simulink model "ELECTRIC_RC_AIRCRAFT_simulink"  (R2025b)
settings: Solver=FixedStepAuto  StartTime=0  StopTime=1000  FixedStep=1/30  RelTol=1e-3
values from neighbouring files (symbols this model uses):
  AoA = [-5 0 5 10 15]    [ELECTRIC_RC_AIRCRAFT.m]
  C_mq = -2*((Tail_Wing_Area/Wing_Surface_Area)*(tail_moment_arm/chord_length_tail))    (= -0.900546448087)    [ELECTRIC_RC_AIRCRAFT.m]
  C_mse = -n*(Tail_Wing_Area/Wing_Surface_Area)*(tail_moment_arm/chord_length_tail)    (= -0.351213114754)    [ELECTRIC_RC_AIRCRAFT.m]
  chord_length = 0.25    [ELECTRIC_RC_AIRCRAFT.m]
  CL = [-0.249 0.205 0.752 1.190 1.316]    [ELECTRIC_RC_AIRCRAFT.m]
  CM = [0.0550 0.0260 -0.0854 -0.1805]    [ELECTRIC_RC_AIRCRAFT.m]
  g = 9.81    [ELECTRIC_RC_AIRCRAFT.m]
  Inertia = (m/12)*(fuselage_length^2+wing_span^2)    (= 0.54883225)    [ELECTRIC_RC_AIRCRAFT.m]
  m = 1.83    [ELECTRIC_RC_AIRCRAFT.m]
  Velocity_initial = 20    [ELECTRIC_RC_AIRCRAFT.m]
  Wing_Surface_Area = 0.4575    [ELECTRIC_RC_AIRCRAFT.m]
libraries: aerolibconvert2 x4, simulink x4, slpidlib x3, aerolibfltsims x2, aerolibadyn x1, aerolibasang x1, aerolibactuator x1, aerolibbdyn x1, aerolibpropulsion2 x1
settings Model: Creator=papar  LastModifiedBy=papar

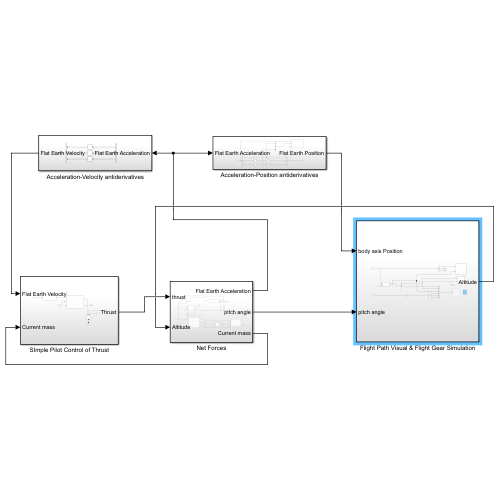
[thumbnail: Simulink's stored preview of the top-level diagram]
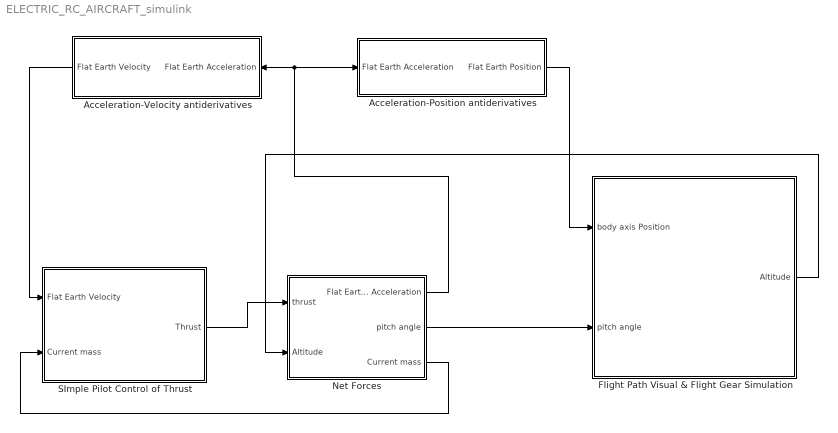
== system ELECTRIC_RC_AIRCRAFT_simulink ==
  Acceleration-Position antiderivatives : Subsystem
  Acceleration-Velocity antiderivatives : Subsystem
  Flight Path Visual & Flight Gear Simulation : Subsystem
  Net Forces : Subsystem
  SImple Pilot Control of Thrust : Subsystem
  wires:
  Acceleration-Velocity antiderivatives/1(Flat Earth Velocity) -> SImple Pilot Control of Thrust/1(Flat Earth Velocity)
  Net Forces/1(Flat Earth Acceleration) -> Acceleration-Velocity antiderivatives/1(Flat Earth Acceleration), Acceleration-Position antiderivatives/1(Flat Earth Acceleration)
  Net Forces/3(Current mass) -> SImple Pilot Control of Thrust/2(Current mass)
  SImple Pilot Control of Thrust/1(Thrust) -> Net Forces/1(thrust)
  Acceleration-Position antiderivatives/1(Flat Earth Position) -> Flight Path Visual & Flight Gear Simulation/1(body axis Position)
  Net Forces/2(pitch angle) -> Flight Path Visual & Flight Gear Simulation/2(pitch angle)
  Flight Path Visual & Flight Gear Simulation/1(Altitude) -> Net Forces/2(Altitude)

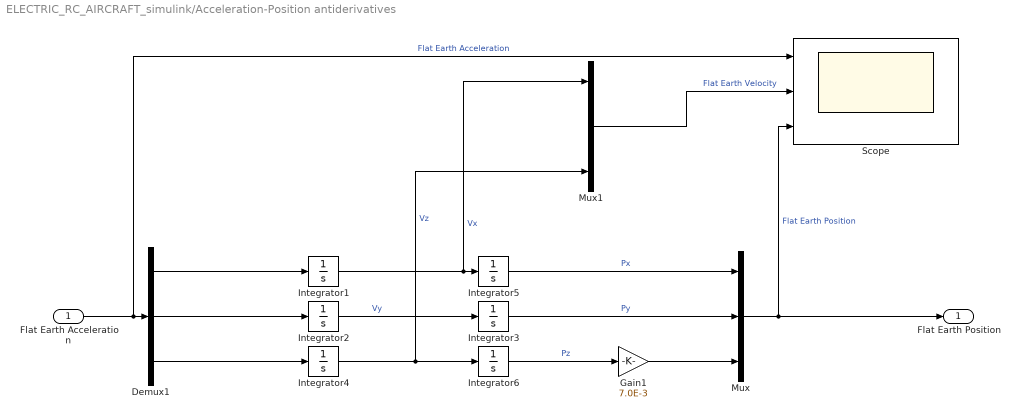
== system ELECTRIC_RC_AIRCRAFT_simulink/Acceleration-Position antiderivatives ==
  Flat Earth Acceleration : Inport
  Demux1 : Demux  Outputs=3
  Gain1 : Gain  Gain=7.0E-3
  Integrator1 : Integrator  InitialCondition=Velocity_initial  UpperSaturationLimit=30  LowerSaturationLimit=-10
  Integrator{2..5} (4 alike) : Integrator
  Integrator6 : Integrator  UpperSaturationLimit=200  LowerSaturationLimit=-100
  Mux : Mux  Inputs=3
  Mux1 : Mux  Inputs=3
  Scope : Scope  NumInputPorts=3
      settings: ActiveDisplayYMinimum=-24.325532445766381  ActiveDisplayYMaximum=34.450960539901729  DataLoggingVariableName=ScopeData2
  Flat Earth Position : Outport
  wires:
  Integrator2/1 -> Integrator3/1  "Vy"
  Flat Earth Acceleration/1 -> Scope/1, Demux1/1  "Flat Earth Acceleration"
  Integrator1/1 -> Mux1/1, Integrator5/1  "Vx"
  Demux1/2 -> Integrator2/1
  Demux1/1 -> Integrator1/1
  Demux1/3 -> Integrator4/1
  Integrator4/1 -> Mux1/3, Integrator6/1  "Vz"
  Mux/1 -> Scope/3, Flat Earth Position/1  "Flat Earth Position"
  Integrator3/1 -> Mux/2  "Py"
  Integrator5/1 -> Mux/1  "Px"
  Integrator6/1 -> Gain1/1  "Pz"
  Gain1/1 -> Mux/3
  Mux1/1 -> Scope/2  "Flat Earth Velocity"

== system ELECTRIC_RC_AIRCRAFT_simulink/Acceleration-Velocity antiderivatives ==
  Flat Earth Acceleration : Inport
  Demux1 : Demux  Outputs=3
  Integrator1 : Integrator
  Integrator2 : Integrator
  Integrator4 : Integrator  InitialCondition=Velocity_initial  UpperSaturationLimit=30  LowerSaturationLimit=-10
  Mux : Mux  Inputs=3
  Flat Earth Velocity : Outport
  wires:
  Mux/1 -> Flat Earth Velocity/1
  Integrator4/1 -> Mux/1  "Vx"
  Demux1/3 -> Integrator1/1
  Demux1/1 -> Integrator4/1
  Demux1/2 -> Integrator2/1
  Integrator1/1 -> Mux/3  "Vz"
  Flat Earth Acceleration/1 -> Demux1/1
  Integrator2/1 -> Mux/2  "Vy"

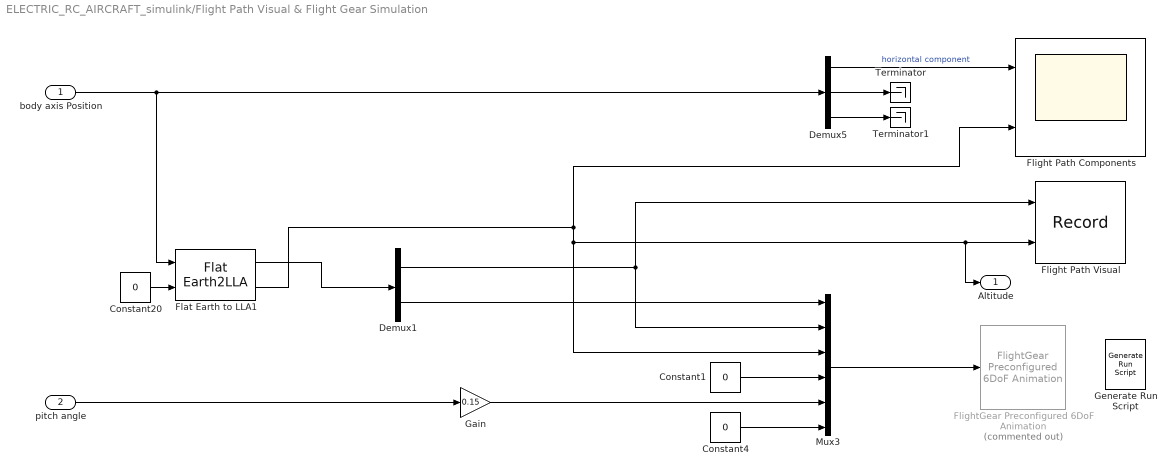
== system ELECTRIC_RC_AIRCRAFT_simulink/Flight Path Visual & Flight Gear Simulation ==
  body axis Position : Inport
  pitch angle : Inport  Port=2
  Constant1 : Constant  Value=0
  Constant20 : Constant  Value=0
  Constant4 : Constant  Value=0
  Demux1 : Demux  Outputs=2
  Demux5 : Demux  Outputs=3
  Flat Earth to LLA1 : FlatEarth2LLA
  Flight Path Components : Scope  NumInputPorts=2
      settings: ActiveDisplayYMinimum=-9.8609130463088863E+6  ActiveDisplayYMaximum=1.5293361483227015E+7
  Flight Path Visual : Record  NumPorts=2.0  FileSettingsInternal="{\"entries\":[{\"content\":{\"excelSettings\":{\"content\":{},\"type\":\"Streamout.ExcelSettings\"},\"parquetSettings\":{\"content\":{},\"type\":\"Streamout.ParquetSettings\"}},\"type\":\"Streamout.FileSettingStorage\",\"uuid\":\"\"}],\"packageUris\":[\"http:\\/\\/schema.mathworks.com\\/mf0\\/streamout_blocks\\/R2020a\"],\"version\":\"1.0\"}"  FrameSettings=[0, 0]  Layout=[1 1]  SignalsInternal="{\"entries\":[{\"content\":{\"signals\":[{\"content\":{\"blockPath\":[],\"dimensions\":[1],\"domain\":\"\",\"lineColor\":\"#a2142f\",\"plots\":[ 1 ],\"port\":1,\"sid\":[\"\"],\"signalID\":1,\"signalName\":\"Demux1:1\"},\"type\":\"RecordBlkView.Signal\",\"uuid\":\"\"},{\"content\":{\"blockPath\":[],\"dimensions\":[1],\"domain\":\"\",\"lineColor\":\"#139fff\",\"plots\":[ 1 ],\"port\":2,\"sid\":[\"\"],\"signalID\":2,\"signalName\":\"Flat Earth to LLA1:2\"},\"type\":\"RecordBlkView.Signal\",\"uuid\":\"\"}]},\"type\":\"RecordBlkView.InputSignals\",\"uuid\":\"\"}],\"packageUris\":[\"http:\\/\\/schema.mathworks.com\\/mf0\\/streamout_blocks\\/R2020a\"],\"version\":\"1.0\"}"  VisualizationBindings="{\"xyplotplugin\":{\"info\":[{\"series\":[{\"bindingParametersList\":[{\"parameter\":\"X-Axis\",\"signalID\":1,\"signalName\":\"Demux1:1\"},{\"parameter\":\"Y-Axis\",\"signalID\":2,\"signalName\":\"Flat Earth to LLA1:2\"}],\"seriesID\":0}],\"subplotID\":1}]}}"  CompatibilityTag=XY
  FlightGear Preconfigured 6DoF Animation : aerolibfltsims/FlightGear Preconfigured 6DoF Animation  Commented=on  xFlightGearVersion=v2019.1  DestinationIpAddress=127.0.0.1  DestinationPort=5502  SampleTime=1/30  packetVersion=24
  Gain : Gain  Gain=0.15
  Generate Run Script : aerolibfltsims/Generate Run Script  Architecture=Win64  dataFlow=Send  GeometryModelName=c172p  AirportId=KSEA  RunwayId=34R  InitialAltitude=0  InitialHeading=0  OffsetDistance=0  OffsetAzimuth=0  InstallScenery=on  DisableShaders=off  OriginAddress=127.0.0.1  DestinationPort=5502  OriginPort=5505  LocalAddress=127.0.0.1  OutputFileName=Final_run.bat  FlightGearBaseDirectory=C:\Program Files\FlightGear 2024.1
  Mux3 : Mux  Inputs=6
  Terminator : Terminator
  Terminator1 : Terminator
  Altitude : Outport
  wires:
  pitch angle/1 -> Gain/1
  Constant1/1 -> Mux3/4
  Flat Earth to LLA1/2 -> Mux3/3, Altitude/1, Flight Path Visual/2, Flight Path Components/2
  Demux5/1 -> Flight Path Components/1  "horizontal component"
  Constant4/1 -> Mux3/6
  Constant20/1 -> Flat Earth to LLA1/2
  Flat Earth to LLA1/1 -> Demux1/1
  Mux3/1 -> FlightGear Preconfigured 6DoF Animation/1
  Demux1/1 -> Flight Path Visual/1, Mux3/2
  body axis Position/1 -> Flat Earth to LLA1/1, Demux5/1
  Demux1/2 -> Mux3/1
  Demux5/3 -> Terminator1/1
  Demux5/2 -> Terminator/1
  Gain/1 -> Mux3/5

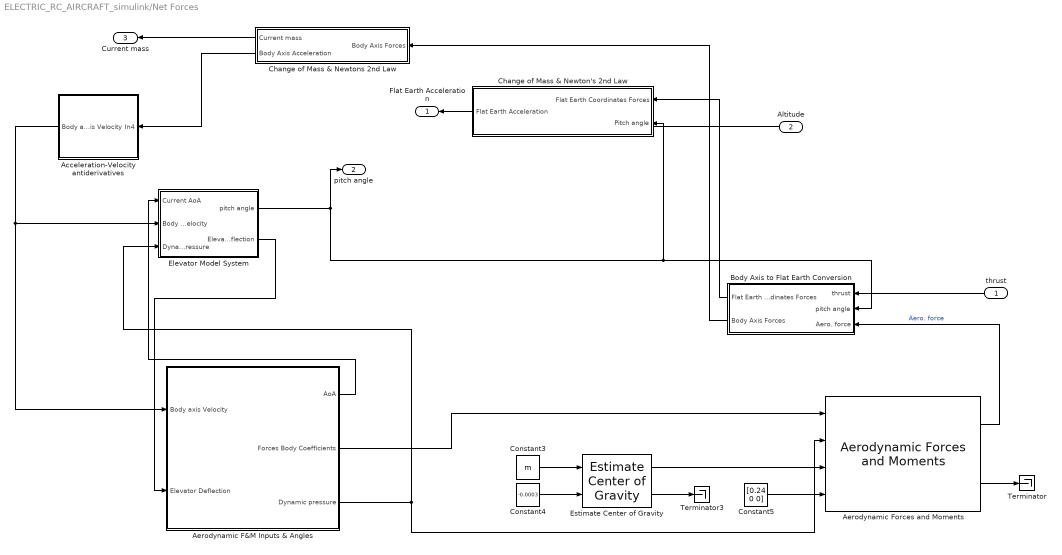
== system ELECTRIC_RC_AIRCRAFT_simulink/Net Forces ==
  thrust : Inport
  Altitude : Inport  Port=2
  Acceleration-Velocity antiderivatives : Subsystem
  "Aerodynamic Forces and Moments " : aerolibadyn/Aerodynamic Forces and Moments   inputAxes=Body  outputForceAxes=Body  outputMomentAxes=Body  S=Wing_Surface_Area  b=1.83  cbar=0.25
  Aerodynamic F&M Inputs & Angles : Subsystem
  Body Axis to Flat Earth Conversion : Subsystem
  Change of Mass & Newton's 2nd Law : Subsystem
  Change of Mass & Newtons 2nd Law : Subsystem
  Constant3 : Constant  Value=m
  Constant4 : Constant  Value=-0.0003
  Constant5 : Constant  Value=[0.24 0 0]
  Elevator Model System : Subsystem
  Estimate Center of Gravity : aerolibbdyn/Estimate Center of Gravity  fmass=m  emass=1.63  fcg=[0.24 0 0]'  ecg=[0.23 0 0]'
  Terminator : Terminator
  Terminator3 : Terminator
  Flat Earth Acceleration : Outport
  pitch angle : Outport  Port=2
  Current mass : Outport  Port=3
  wires:
  Constant5/1 -> "Aerodynamic Forces and Moments "/4
  Estimate Center of Gravity/1 -> "Aerodynamic Forces and Moments "/3
  Acceleration-Velocity antiderivatives/1(Body axis Velocity) -> Aerodynamic F&M Inputs & Angles/1(Body axis Velocity), Elevator Model System/2(Body axis Velocity)
  Constant3/1 -> Estimate Center of Gravity/1
  Constant4/1 -> Estimate Center of Gravity/2
  "Aerodynamic Forces and Moments "/2 -> Terminator/1
  Estimate Center of Gravity/2 -> Terminator3/1
  Aerodynamic F&M Inputs & Angles/3(Dynamic pressure) -> "Aerodynamic Forces and Moments "/2, Elevator Model System/3(Dynamic pressure)
  Aerodynamic F&M Inputs & Angles/2(Forces Body Coefficients) -> "Aerodynamic Forces and Moments "/1
  Aerodynamic F&M Inputs & Angles/1(AoA) -> Elevator Model System/1(Current AoA)
  Change of Mass & Newtons 2nd Law/1(Current mass) -> Current mass/1
  Change of Mass & Newtons 2nd Law/2(Body Axis Acceleration) -> Acceleration-Velocity antiderivatives/1(In4)
  Change of Mass & Newton's 2nd Law/1(Flat Earth Acceleration) -> Flat Earth Acceleration/1
  thrust/1 -> Body Axis to Flat Earth Conversion/1(thrust)
  Elevator Model System/1(pitch angle) -> Change of Mass & Newton's 2nd Law/2(Pitch angle), Body Axis to Flat Earth Conversion/2(pitch angle), pitch angle/1
  "Aerodynamic Forces and Moments "/1 -> Body Axis to Flat Earth Conversion/3(Aero. force)  "Aero. force"
  Body Axis to Flat Earth Conversion/1(Flat Earth Coordinates Forces) -> Change of Mass & Newton's 2nd Law/1(Flat Earth Coordinates Forces)
  Body Axis to Flat Earth Conversion/2(Body Axis Forces) -> Change of Mass & Newtons 2nd Law/1(Body Axis Forces)
  Elevator Model System/2(Elevator Deflection) -> Aerodynamic F&M Inputs & Angles/2(Elevator Deflection)
  Altitude/1 -> ?

== system ELECTRIC_RC_AIRCRAFT_simulink/SImple Pilot Control of Thrust ==
  Flat Earth Velocity : Inport
  Current mass : Inport  Port=2
  Constant2 : Constant  Value=0
  Constant3 : Constant  Value=0.05
  Constant5 : Constant  Value=0
  Simple Autopilot : Subsystem
  Switch : Switch  Criteria=u2 > Threshold  Threshold=1.63  SaturateOnIntegerOverflow=off  InputSameDT=off
  Terminator2 : Terminator
  Turbofan Engine System : aerolibpropulsion2/Turbofan Engine System  units=Metric (MKS)  ic_source=Internal  IC=30  Fmax=30  tau=0.4  SFC=0  Nt=0.9
  Thrust : Outport
  wires:
  Simple Autopilot/1(current throttle) -> Turbofan Engine System/1
  Constant3/1 -> Turbofan Engine System/2
  Constant5/1 -> Switch/3
  Turbofan Engine System/1 -> Switch/1  "thrust"
  Constant2/1 -> Turbofan Engine System/3
  Current mass/1 -> Switch/2
  Flat Earth Velocity/1 -> Simple Autopilot/1(body axis velocity)
  Switch/1 -> Thrust/1
  Turbofan Engine System/2 -> Terminator2/1

== system ELECTRIC_RC_AIRCRAFT_simulink/Net Forces/Acceleration-Velocity antiderivatives ==
  In4 : Inport
  Demux1 : Demux  Outputs=3
  Integrator1 : Integrator
  Integrator2 : Integrator
  Integrator4 : Integrator  InitialCondition=Velocity_initial  UpperSaturationLimit=30  LowerSaturationLimit=-10
  Mux : Mux  Inputs=3
  Body axis Velocity : Outport
  wires:
  Integrator2/1 -> Mux/2  "Vy"
  In4/1 -> Demux1/1
  Integrator1/1 -> Mux/3  "Vz"
  Demux1/2 -> Integrator2/1
  Demux1/1 -> Integrator4/1
  Demux1/3 -> Integrator1/1
  Integrator4/1 -> Mux/1  "Vx"
  Mux/1 -> Body axis Velocity/1

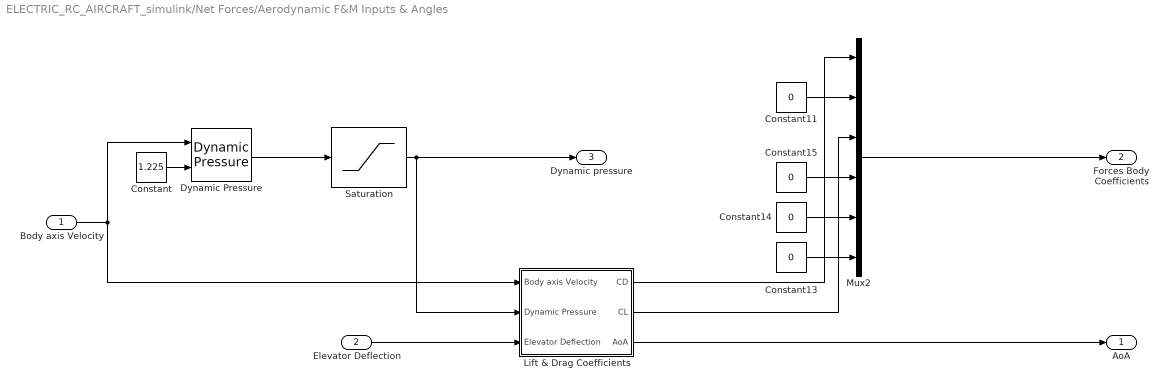
== system ELECTRIC_RC_AIRCRAFT_simulink/Net Forces/Aerodynamic F&M Inputs & Angles ==
  Body axis Velocity : Inport
  Elevator Deflection : Inport  Port=2
  Constant : Constant  Value=1.225
  Constant{11,13..15} (4 alike) : Constant  Value=0
  Dynamic Pressure : aerolibasang/Dynamic Pressure
  Lift & Drag Coefficients : Subsystem
  Mux2 : Mux  Inputs=6
  Saturation : Saturate  UpperLimit=200  LowerLimit=0  LinearizeAsGain=off
  AoA : Outport
  Forces Body Coefficients : Outport  Port=2
  Dynamic pressure : Outport  Port=3
  wires:
  Constant/1 -> Dynamic Pressure/2
  Lift & Drag Coefficients/2(CL) -> Mux2/3
  Body axis Velocity/1 -> Dynamic Pressure/1, Lift & Drag Coefficients/1(Body axis Velocity)
  Constant11/1 -> Mux2/2
  Constant14/1 -> Mux2/5
  Constant13/1 -> Mux2/6
  Dynamic Pressure/1 -> Saturation/1
  Constant15/1 -> Mux2/4
  Lift & Drag Coefficients/1(CD) -> Mux2/1
  Elevator Deflection/1 -> Lift & Drag Coefficients/3(Elevator Deflection)
  Lift & Drag Coefficients/3(AoA) -> AoA/1
  Mux2/1 -> Forces Body Coefficients/1
  Saturation/1 -> Lift & Drag Coefficients/2(Dynamic Pressure), Dynamic pressure/1

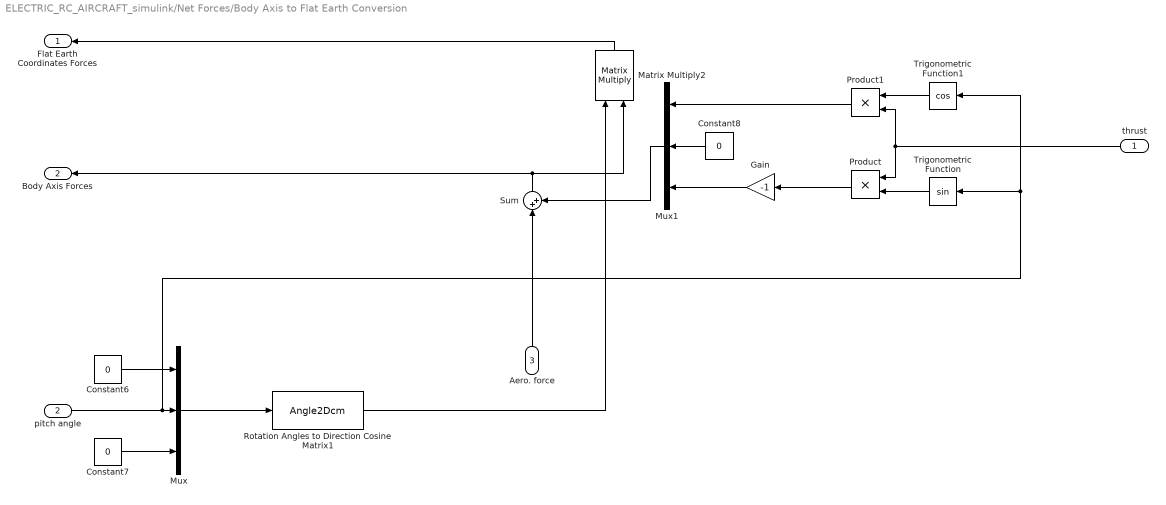
== system ELECTRIC_RC_AIRCRAFT_simulink/Net Forces/Body Axis to Flat Earth Conversion ==
  thrust : Inport
  pitch angle : Inport  Port=2
  Aero. force : Inport  Port=3
  Constant6 : Constant  Value=0
  Constant7 : Constant  Value=0
  Constant8 : Constant  Value=0
  Gain : Gain  Gain=-1
  Matrix Multiply2 : Product  Multiplication=Matrix(*)
  Mux : Mux  Inputs=3
  Mux1 : Mux  Inputs=3
  Product : Product
  Product1 : Product
  Rotation Angles to Direction Cosine Matrix1 : Angle2Dcm  rotationOrder=XYZ
      settings: AttributesFormatString=Rotation Order: %<rotationOrder>
  Sum : Sum  Inputs=|++
  Trigonometric Function : Trigonometry
  Trigonometric Function1 : Trigonometry  Operator=cos
  Flat Earth Coordinates Forces : Outport
  Body Axis Forces : Outport  Port=2
  wires:
  Constant7/1 -> Mux/3
  pitch angle/1 -> Trigonometric Function1/1, Trigonometric Function/1, Mux/2
  Sum/1 -> Body Axis Forces/1, Matrix Multiply2/2
  Product/1 -> Gain/1
  Constant6/1 -> Mux/1
  thrust/1 -> Product1/2, Product/1
  Constant8/1 -> Mux1/2
  Mux1/1 -> Sum/2
  Mux/1 -> Rotation Angles to Direction Cosine Matrix1/1
  Rotation Angles to Direction Cosine Matrix1/1 -> Matrix Multiply2/1
  Matrix Multiply2/1 -> Flat Earth Coordinates Forces/1
  Aero. force/1 -> Sum/1
  Trigonometric Function/1 -> Product/2
  Trigonometric Function1/1 -> Product1/1
  Product1/1 -> Mux1/1
  Gain/1 -> Mux1/3

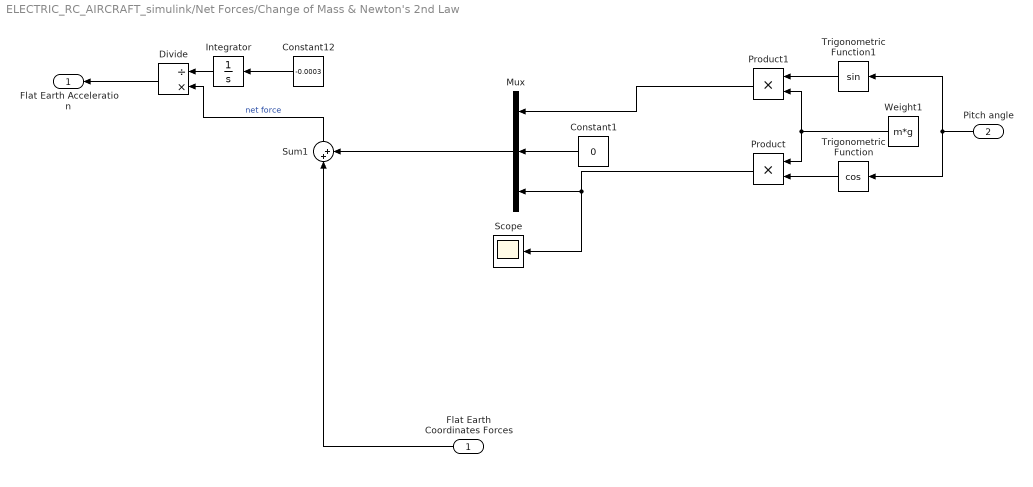
== system ELECTRIC_RC_AIRCRAFT_simulink/Net Forces/Change of Mass & Newton's 2nd Law ==
  Flat Earth Coordinates Forces : Inport
  Pitch angle : Inport  Port=2
  Constant1 : Constant  Value=0
  Constant12 : Constant  Value=-0.0003
  Divide : Product  Inputs=/*
  Integrator : Integrator  InitialCondition=m  LimitOutput=on  UpperSaturationLimit=1.83  LowerSaturationLimit=1.63
  Mux : Mux  Inputs=3
  Product : Product
  Product1 : Product
  Scope : Scope
      settings: ActiveDisplayYMinimum=-299.86450667142719  ActiveDisplayYMaximum=328.98932299890214
  Sum1 : Sum  Inputs=|++
  Trigonometric Function : Trigonometry  Operator=cos
  Trigonometric Function1 : Trigonometry
  Weight1 : Constant  Value=m*g
  Flat Earth Acceleration : Outport
  wires:
  Constant12/1 -> Integrator/1
  Divide/1 -> Flat Earth Acceleration/1
  Sum1/1 -> Divide/2  "net force"
  Flat Earth Coordinates Forces/1 -> Sum1/1
  Integrator/1 -> Divide/1
  Weight1/1 -> Product1/2, Product/1
  Trigonometric Function/1 -> Product/2
  Trigonometric Function1/1 -> Product1/1
  Product1/1 -> Mux/1
  Pitch angle/1 -> Trigonometric Function/1, Trigonometric Function1/1
  Mux/1 -> Sum1/2
  Constant1/1 -> Mux/2
  Product/1 -> Scope/1, Mux/3

== system ELECTRIC_RC_AIRCRAFT_simulink/Net Forces/Change of Mass & Newtons 2nd Law ==
  Body Axis Forces : Inport
  Constant2 : Constant  Value=-0.0003
  Divide1 : Product  Inputs=/*
  Integrator1 : Integrator  InitialCondition=m  LimitOutput=on  UpperSaturationLimit=1.83  LowerSaturationLimit=1.63
  Sum3 : Sum  Inputs=|++
  Weight2 : Constant  Value=[0 0 m*g]
  Current mass : Outport
  Body Axis Acceleration : Outport  Port=2
  wires:
  Constant2/1 -> Integrator1/1
  Sum3/1 -> Divide1/2  "net force"
  Divide1/1 -> Body Axis Acceleration/1
  Weight2/1 -> Sum3/2
  Body Axis Forces/1 -> Sum3/1
  Integrator1/1 -> Divide1/1, Current mass/1

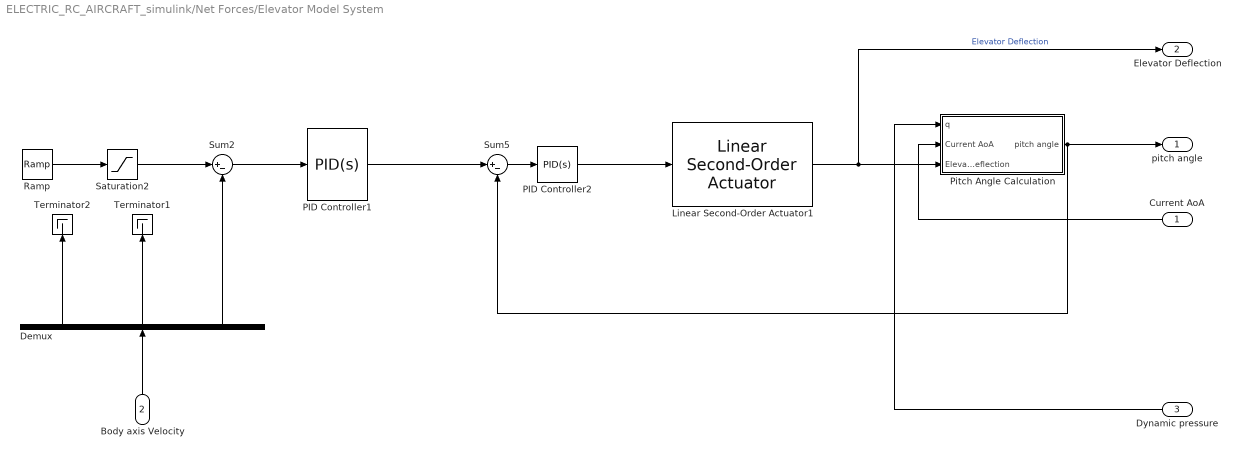
== system ELECTRIC_RC_AIRCRAFT_simulink/Net Forces/Elevator Model System ==
  Current AoA : Inport
  Body axis Velocity : Inport  Port=2
  Dynamic pressure : Inport  Port=3
  Demux : Demux  Outputs=3
  Linear Second-Order Actuator1 : aerolibactuator/Linear Second-Order Actuator  wn_fin=8  z_fin=0.7  fin_act_0=0  fin_act_vel=0
  PID Controller1 : slpidlib/PID Controller  Controller=PID  Form=Parallel  TimeDomain=Continuous-time  UseExternalTs=off  SampleTime=-1  IntegratorMethod=Forward Euler  FilterMethod=Forward Euler  ControllerParametersSource=internal  P=0.5  I=0  UseKiTs=off  D=0.5  UseExternalDerivativeSource=off  N=10  UseFilter=on  TunerSelectOption=Transfer Function Based (PID Tuner App)  InitialConditionSource=internal  InitialConditionForIntegrator=0  InitialConditionForFilter=0  DifferentiatorICPrevScaledInput=0  ExternalReset=none  TrackingMode=off  Kt=1  LimitOutput=off  SatLimitsSource=internal  UpperSaturationLimit=0.17  LowerSaturationLimit=-0.17  LinearizeAsGain=on  AntiWindupMode=clamping  Kb=1  LimitIntegrator=off  UpperIntegratorSaturationLimit=inf  LowerIntegratorSaturationLimit=-inf  POutMin=[]  POutMax=[]  IOutMin=[]  IOutMax=[]  DOutMin=[]  DOutMax=[]  NOutMin=[]  NOutMax=[]  SumOutMin=[]  SumOutMax=[]  SaturationOutMin=[]  SaturationOutMax=[]  PParamMin=[]  PParamMax=[]  IParamMin=[]  IParamMax=[]  DParamMin=[]  DParamMax=[]  NParamMin=[]  NParamMax=[]  KbParamMin=[]  KbParamMax=[]  KtParamMin=[]  KtParamMax=[]  KbOutMin=[]  KbOutMax=[]  KtOutMin=[]  KtOutMax=[]  IntegratorOutMin=[]  IntegratorOutMax=[]  FilterOutMin=[]  FilterOutMax=[]  SumI1OutMin=[]  SumI1OutMax=[]  SumI2OutMin=[]  SumI2OutMax=[]  SumI3OutMin=[]  SumI3OutMax=[]  SumI4OutMin=[]  SumI4OutMax=[]  SumDOutMin=[]  SumDOutMax=[]  DifferentiatorOutMin=[]  DifferentiatorOutMax=[]  FilterDiffOutCoefMin=[]  FilterDiffOutCoefMax=[]  ReciprocalOutMin=[]  ReciprocalOutMax=[]  SumDenOutMin=[]  SumDenOutMax=[]  SumNumOutMin=[]  SumNumOutMax=[]  DivideOutMin=[]  DivideOutMax=[]  UdiffTsProdOutMin=[]  UdiffTsProdOutMax=[]  NTsProdOutMin=[]  NTsProdOutMax=[]  UintegralTsProdOutMin=[]  UintegralTsProdOutMax=[]  UngainTsProdOutMin=[]  UngainTsProdOutMax=[]  ClampingZeroOutDataTypeStr=Inherit: Inherit via back propagation  ClampingZeroOutMin=[]  ClampingZeroOutMax=[]  FilterDenConstantOutDataTypeStr=Inherit: Inherit via back propagation  FilterDenConstantOutMin=[]  FilterDenConstantOutMax=[]  PCopyOutDataTypeStr=Inherit: Inherit via back propagation  PCopyOutMin=[]  PCopyOutMax=[]  NCopyOutDataTypeStr=Inherit: Inherit via back propagation  NCopyOutMin=[]  NCopyOutMax=[]  IntegratorContinuousStateAttributes=''  IntegratorStateMustResolveToSignalObject=off  IntegratorRTWStateStorageClass=Auto  FilterContinuousStateAttributes=''  FilterStateMustResolveToSignalObject=off  FilterRTWStateStorageClass=Auto  ParallelPVariant=InternalParameters  IdealPVariant=Disabled  IVariant=InternalParameters  DVariant=InternalParameters  IntegratorVariant=Continuous  SatVariant=Disabled  AWVariant=Passthrough  PCopyVariant=Disabled  TRVariant=Disabled  FdbkBlocksVariant=Forward  IdealPFdbkVariant=Disabled  SatFdbkVariant=Disabled  DerivativeFilterVariant=ContFilter  NVariant=InternalParameters  NCopyVariant=Disabled  FilterICVariant=InternalICsFilter  IntegratorICVariant=InternalICs  ExternalResetVariant=Disabled  TRSumVariant=Passthrough  SumFdbkVariant=Disabled  SumVariant=Sum_PID  TsampFilterVariant=InternalTs  TsampNgainVariant=Passthrough  TsampIntegralVariant=Disabled_SignalSpec  ExternalSaturationOutDataTypeStr=Inherit: Same as second input  DerivativeSourceVariant=ErrorSignal  PreIntVariant=InternalPreInt
  PID Controller2 : slpidlib/PID Controller  Controller=PID  Form=Parallel  TimeDomain=Continuous-time  UseExternalTs=off  SampleTime=-1  IntegratorMethod=Forward Euler  FilterMethod=Forward Euler  ControllerParametersSource=internal  P=1.0E-3  I=0  UseKiTs=off  D=1.0E-3  UseExternalDerivativeSource=off  N=20  UseFilter=on  TunerSelectOption=Transfer Function Based (PID Tuner App)  InitialConditionSource=internal  InitialConditionForIntegrator=0  InitialConditionForFilter=0  DifferentiatorICPrevScaledInput=0  ExternalReset=none  TrackingMode=off  Kt=1  LimitOutput=off  SatLimitsSource=internal  UpperSaturationLimit=inf  LowerSaturationLimit=-inf  LinearizeAsGain=on  AntiWindupMode=none  Kb=1  LimitIntegrator=off  UpperIntegratorSaturationLimit=inf  LowerIntegratorSaturationLimit=-inf  POutMin=[]  POutMax=[]  IOutMin=[]  IOutMax=[]  DOutMin=[]  DOutMax=[]  NOutMin=[]  NOutMax=[]  SumOutMin=[]  SumOutMax=[]  SaturationOutMin=[]  SaturationOutMax=[]  PParamMin=[]  PParamMax=[]  IParamMin=[]  IParamMax=[]  DParamMin=[]  DParamMax=[]  NParamMin=[]  NParamMax=[]  KbParamMin=[]  KbParamMax=[]  KtParamMin=[]  KtParamMax=[]  KbOutMin=[]  KbOutMax=[]  KtOutMin=[]  KtOutMax=[]  IntegratorOutMin=[]  IntegratorOutMax=[]  FilterOutMin=[]  FilterOutMax=[]  SumI1OutMin=[]  SumI1OutMax=[]  SumI2OutMin=[]  SumI2OutMax=[]  SumI3OutMin=[]  SumI3OutMax=[]  SumI4OutMin=[]  SumI4OutMax=[]  SumDOutMin=[]  SumDOutMax=[]  DifferentiatorOutMin=[]  DifferentiatorOutMax=[]  FilterDiffOutCoefMin=[]  FilterDiffOutCoefMax=[]  ReciprocalOutMin=[]  ReciprocalOutMax=[]  SumDenOutMin=[]  SumDenOutMax=[]  SumNumOutMin=[]  SumNumOutMax=[]  DivideOutMin=[]  DivideOutMax=[]  UdiffTsProdOutMin=[]  UdiffTsProdOutMax=[]  NTsProdOutMin=[]  NTsProdOutMax=[]  UintegralTsProdOutMin=[]  UintegralTsProdOutMax=[]  UngainTsProdOutMin=[]  UngainTsProdOutMax=[]  ClampingZeroOutDataTypeStr=Inherit: Inherit via back propagation  ClampingZeroOutMin=[]  ClampingZeroOutMax=[]  FilterDenConstantOutDataTypeStr=Inherit: Inherit via back propagation  FilterDenConstantOutMin=[]  FilterDenConstantOutMax=[]  PCopyOutDataTypeStr=Inherit: Inherit via back propagation  PCopyOutMin=[]  PCopyOutMax=[]  NCopyOutDataTypeStr=Inherit: Inherit via back propagation  NCopyOutMin=[]  NCopyOutMax=[]  IntegratorContinuousStateAttributes=''  IntegratorStateMustResolveToSignalObject=off  IntegratorRTWStateStorageClass=Auto  FilterContinuousStateAttributes=''  FilterStateMustResolveToSignalObject=off  FilterRTWStateStorageClass=Auto  ParallelPVariant=InternalParameters  IdealPVariant=Disabled  IVariant=InternalParameters  DVariant=InternalParameters  IntegratorVariant=Continuous  SatVariant=Disabled  AWVariant=Passthrough  PCopyVariant=Disabled  TRVariant=Disabled  FdbkBlocksVariant=Forward  IdealPFdbkVariant=Disabled  SatFdbkVariant=Disabled  DerivativeFilterVariant=ContFilter  NVariant=InternalParameters  NCopyVariant=Disabled  FilterICVariant=InternalICsFilter  IntegratorICVariant=InternalICs  ExternalResetVariant=Disabled  TRSumVariant=Passthrough  SumFdbkVariant=Disabled  SumVariant=Sum_PID  TsampFilterVariant=InternalTs  TsampNgainVariant=Passthrough  TsampIntegralVariant=Disabled_SignalSpec  ExternalSaturationOutDataTypeStr=Inherit: Same as second input  DerivativeSourceVariant=ErrorSignal  PreIntVariant=InternalPreInt
  Pitch Angle Calculation : Subsystem
  Ramp : simulink/Sources/Ramp  slope=-1.0E-1  start=0  InitialOutput=0
  Saturation2 : Saturate  UpperLimit=0  LowerLimit=-200
  Sum2 : Sum  Inputs=|+-
  Sum5 : Sum  Inputs=|+-
  Terminator1 : Terminator
  Terminator2 : Terminator
  pitch angle : Outport
  Elevator Deflection : Outport  Port=2
  wires:
  Ramp/1 -> Saturation2/1
  PID Controller2/1 -> Linear Second-Order Actuator1/1
  Demux/3 -> Sum2/2
  Dynamic pressure/1 -> Pitch Angle Calculation/1(q)
  Pitch Angle Calculation/1(pitch angle) -> Sum5/2, pitch angle/1
  Saturation2/1 -> Sum2/1
  Linear Second-Order Actuator1/1 -> Elevator Deflection/1, Pitch Angle Calculation/3(Elevator Deflection)  "Elevator Deflection"
  Sum5/1 -> PID Controller2/1
  PID Controller1/1 -> Sum5/1
  Sum2/1 -> PID Controller1/1
  Demux/2 -> Terminator1/1
  Demux/1 -> Terminator2/1
  Current AoA/1 -> Pitch Angle Calculation/2(Current AoA)
  Body axis Velocity/1 -> Demux/1

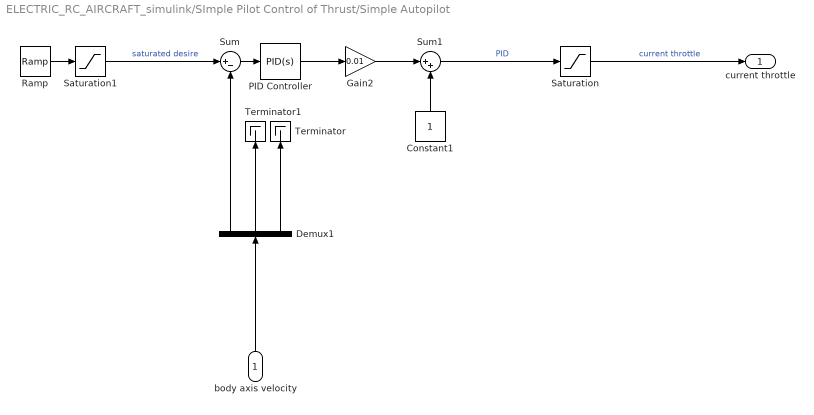
== system ELECTRIC_RC_AIRCRAFT_simulink/SImple Pilot Control of Thrust/Simple Autopilot ==
  body axis velocity : Inport
  Constant1 : Constant
  Demux1 : Demux  Outputs=3
  Gain2 : Gain  Gain=0.01
  PID Controller : slpidlib/PID Controller  Controller=PID  Form=Parallel  TimeDomain=Continuous-time  UseExternalTs=off  SampleTime=-1  IntegratorMethod=Forward Euler  FilterMethod=Forward Euler  ControllerParametersSource=internal  P=0.5  I=5.0E-3  UseKiTs=off  D=0.1  UseExternalDerivativeSource=off  N=20  UseFilter=on  TunerSelectOption=Transfer Function Based (PID Tuner App)  InitialConditionSource=internal  InitialConditionForIntegrator=0  InitialConditionForFilter=0  DifferentiatorICPrevScaledInput=0  ExternalReset=none  TrackingMode=off  Kt=1  LimitOutput=off  SatLimitsSource=internal  UpperSaturationLimit=inf  LowerSaturationLimit=-inf  LinearizeAsGain=on  AntiWindupMode=none  Kb=1  LimitIntegrator=off  UpperIntegratorSaturationLimit=inf  LowerIntegratorSaturationLimit=-inf  POutMin=[]  POutMax=[]  IOutMin=[]  IOutMax=[]  DOutMin=[]  DOutMax=[]  NOutMin=[]  NOutMax=[]  SumOutMin=[]  SumOutMax=[]  SaturationOutMin=[]  SaturationOutMax=[]  PParamMin=[]  PParamMax=[]  IParamMin=[]  IParamMax=[]  DParamMin=[]  DParamMax=[]  NParamMin=[]  NParamMax=[]  KbParamMin=[]  KbParamMax=[]  KtParamMin=[]  KtParamMax=[]  KbOutMin=[]  KbOutMax=[]  KtOutMin=[]  KtOutMax=[]  IntegratorOutMin=[]  IntegratorOutMax=[]  FilterOutMin=[]  FilterOutMax=[]  SumI1OutMin=[]  SumI1OutMax=[]  SumI2OutMin=[]  SumI2OutMax=[]  SumI3OutMin=[]  SumI3OutMax=[]  SumI4OutMin=[]  SumI4OutMax=[]  SumDOutMin=[]  SumDOutMax=[]  DifferentiatorOutMin=[]  DifferentiatorOutMax=[]  FilterDiffOutCoefMin=[]  FilterDiffOutCoefMax=[]  ReciprocalOutMin=[]  ReciprocalOutMax=[]  SumDenOutMin=[]  SumDenOutMax=[]  SumNumOutMin=[]  SumNumOutMax=[]  DivideOutMin=[]  DivideOutMax=[]  UdiffTsProdOutMin=[]  UdiffTsProdOutMax=[]  NTsProdOutMin=[]  NTsProdOutMax=[]  UintegralTsProdOutMin=[]  UintegralTsProdOutMax=[]  UngainTsProdOutMin=[]  UngainTsProdOutMax=[]  ClampingZeroOutDataTypeStr=Inherit: Inherit via back propagation  ClampingZeroOutMin=[]  ClampingZeroOutMax=[]  FilterDenConstantOutDataTypeStr=Inherit: Inherit via back propagation  FilterDenConstantOutMin=[]  FilterDenConstantOutMax=[]  PCopyOutDataTypeStr=Inherit: Inherit via back propagation  PCopyOutMin=[]  PCopyOutMax=[]  NCopyOutDataTypeStr=Inherit: Inherit via back propagation  NCopyOutMin=[]  NCopyOutMax=[]  IntegratorContinuousStateAttributes=''  IntegratorStateMustResolveToSignalObject=off  IntegratorRTWStateStorageClass=Auto  FilterContinuousStateAttributes=''  FilterStateMustResolveToSignalObject=off  FilterRTWStateStorageClass=Auto  ParallelPVariant=InternalParameters  IdealPVariant=Disabled  IVariant=InternalParameters  DVariant=InternalParameters  IntegratorVariant=Continuous  SatVariant=Disabled  AWVariant=Passthrough  PCopyVariant=Disabled  TRVariant=Disabled  FdbkBlocksVariant=Forward  IdealPFdbkVariant=Disabled  SatFdbkVariant=Disabled  DerivativeFilterVariant=ContFilter  NVariant=InternalParameters  NCopyVariant=Disabled  FilterICVariant=InternalICsFilter  IntegratorICVariant=InternalICs  ExternalResetVariant=Disabled  TRSumVariant=Passthrough  SumFdbkVariant=Disabled  SumVariant=Sum_PID  TsampFilterVariant=InternalTs  TsampNgainVariant=Passthrough  TsampIntegralVariant=Disabled_SignalSpec  ExternalSaturationOutDataTypeStr=Inherit: Same as second input  DerivativeSourceVariant=ErrorSignal  PreIntVariant=InternalPreInt
  Ramp : simulink/Sources/Ramp  slope=-3.0E-2  start=0  InitialOutput=7
  Saturation : Saturate  UpperLimit=1  LowerLimit=0  LinearizeAsGain=off
  Saturation1 : Saturate  UpperLimit=7  LowerLimit=4  LinearizeAsGain=off
  Sum : Sum  Inputs=|+-
  Sum1 : Sum  Inputs=|++
  Terminator : Terminator
  Terminator1 : Terminator
  current throttle : Outport
  wires:
  Ramp/1 -> Saturation1/1
  Sum1/1 -> Saturation/1  "PID"
  Constant1/1 -> Sum1/2
  Gain2/1 -> Sum1/1
  Demux1/1 -> Sum/2
  Saturation1/1 -> Sum/1  "saturated desire"
  Saturation/1 -> current throttle/1  "current throttle"
  PID Controller/1 -> Gain2/1
  Sum/1 -> PID Controller/1
  body axis velocity/1 -> Demux1/1
  Demux1/2 -> Terminator1/1
  Demux1/3 -> Terminator/1

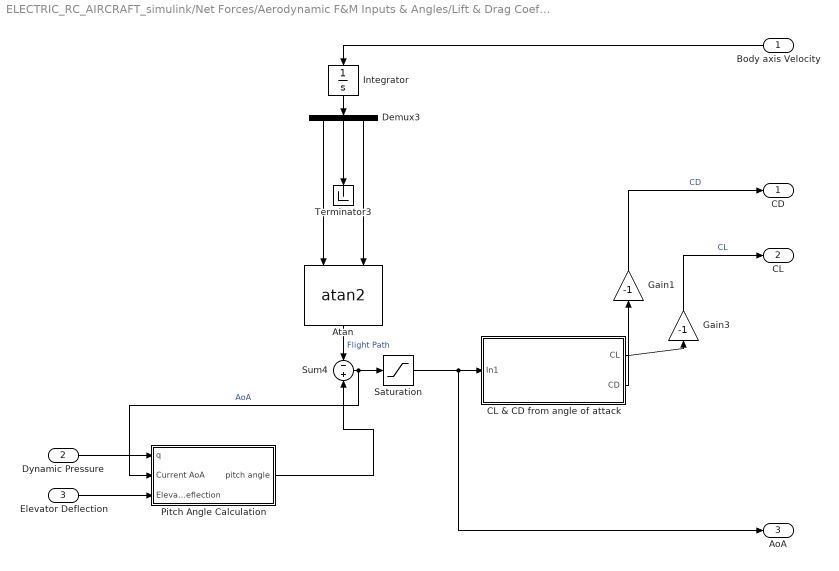
== system ELECTRIC_RC_AIRCRAFT_simulink/Net Forces/Aerodynamic F&M Inputs & Angles/Lift & Drag Coefficients ==
  Body axis Velocity : Inport
  Dynamic Pressure : Inport  Port=2
  Elevator Deflection : Inport  Port=3
  Atan : Trigonometry  Operator=atan2
  CL & CD from angle of attack : Subsystem
  Demux3 : Demux  Outputs=3
  Gain1 : Gain  Gain=-1
  Gain3 : Gain  Gain=-1
  Integrator : Integrator
  Pitch Angle Calculation : Subsystem
  Saturation : Saturate  UpperLimit=2  LowerLimit=-2  LinearizeAsGain=off
  Sum4 : Sum  Inputs=-+
  Terminator3 : Terminator
  CD : Outport
  CL : Outport  Port=2
  AoA : Outport  Port=3
  wires:
  Gain3/1 -> CL/1  "CL"
  Demux3/3 -> Atan/2
  CL & CD from angle of attack/1(CL) -> Gain3/1
  Atan/1 -> Sum4/1  "Flight Path"
  Demux3/1 -> Atan/1
  Sum4/1 -> Pitch Angle Calculation/2(Current AoA), Saturation/1  "AoA"
  CL & CD from angle of attack/2(CD) -> Gain1/1
  Dynamic Pressure/1 -> Pitch Angle Calculation/1(q)
  Gain1/1 -> CD/1  "CD"
  Saturation/1 -> AoA/1, CL & CD from angle of attack/1(In1)
  Elevator Deflection/1 -> Pitch Angle Calculation/3(Elevator Deflection)
  Pitch Angle Calculation/1(pitch angle) -> Sum4/2
  Integrator/1 -> Demux3/1
  Body axis Velocity/1 -> Integrator/1
  Demux3/2 -> Terminator3/1

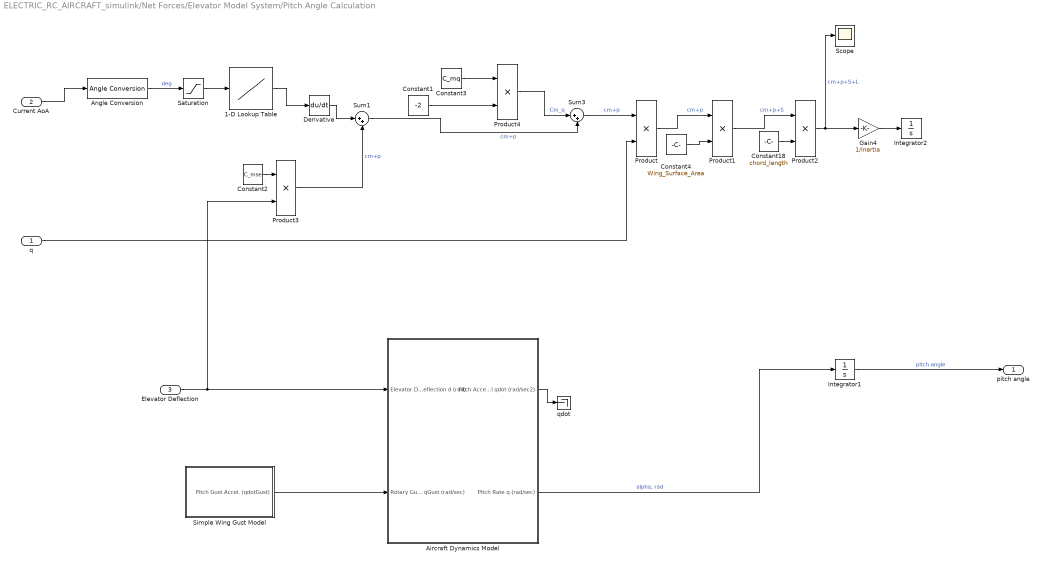
== system ELECTRIC_RC_AIRCRAFT_simulink/Net Forces/Elevator Model System/Pitch Angle Calculation ==
  q : Inport
  Current AoA : Inport  Port=2
  Elevator Deflection : Inport  Port=3
  1-D Lookup Table : Lookup_n-D  NumberOfTableDimensions=1  BreakpointsForDimension1=[-5 0 5 10]  Table=CM  InternalRulePriority=Speed  RndMeth=Simplest
  Aircraft Dynamics Model : Subsystem
  Angle Conversion : aerolibconvert2/Angle Conversion  IU=rad  OU=deg
  Constant1 : Constant  Value=-2
  Constant18 : Constant  Value=chord_length
  Constant2 : Constant  Value=C_mse
  Constant3 : Constant  Value=C_mq
  Constant4 : Constant  Value=Wing_Surface_Area
  Derivative : Derivative
  Gain4 : Gain  Gain=1/Inertia
  Integrator1 : Integrator
  Integrator2 : Integrator
  Product{,1..4} (5 alike) : Product
  Saturation : Saturate  UpperLimit=10  LowerLimit=-10  LinearizeAsGain=off
  Scope : Scope
      settings: ActiveDisplayYMinimum=-2.2976167129136656E+27  ActiveDisplayYMaximum=2.0678550416222997E+28  DataLoggingVariableName=ScopeData5
  Simple Wing Gust Model : Subsystem
  Sum1 : Sum  Inputs=|++
  Sum3 : Sum  Inputs=|++
  qdot : Terminator
  pitch angle : Outport
  wires:
  Product/1 -> Product1/1  "cm+p"
  Constant18/1 -> Product2/2
  Product1/1 -> Product2/1  "cm+p+S"
  Current AoA/1 -> Angle Conversion/1
  Constant4/1 -> Product1/2
  Gain4/1 -> Integrator2/1
  Saturation/1 -> 1-D Lookup Table/1
  Product2/1 -> Scope/1, Gain4/1  "cm+p+S+L"
  Angle Conversion/1 -> Saturation/1  "deg"
  1-D Lookup Table/1 -> Derivative/1
  Derivative/1 -> Sum1/1
  Sum1/1 -> Sum3/2  "cm+p"
  Elevator Deflection/1 -> Product3/2, Aircraft Dynamics Model/1(Elevator Deflection d (rad))
  Constant1/1 -> Product4/2
  Product4/1 -> Sum3/1  "Cm_q"
  Constant2/1 -> Product3/1
  Product3/1 -> Sum1/2  "cm+p"
  Constant3/1 -> Product4/1
  Sum3/1 -> Product/1  "cm+p"
  Integrator1/1 -> pitch angle/1  "pitch angle"
  Aircraft Dynamics Model/1(Pitch Accel qdot (rad/sec2)) -> qdot/1
  q/1 -> Product/2
  Aircraft Dynamics Model/2(Pitch Rate q (rad/sec)) -> Integrator1/1  "alpha, rad"
  Simple Wing Gust Model/1(Pitch Gust Accel. (qdotGust)) -> Aircraft Dynamics Model/2(Rotary Gust qGust (rad/sec))

== system ELECTRIC_RC_AIRCRAFT_simulink/Net Forces/Aerodynamic F&M Inputs & Angles/Lift & Drag Coefficients/CL & CD from angle of attack ==
  In1 : Inport
  1-D Lookup Table : Lookup_n-D  NumberOfTableDimensions=1  BreakpointsForDimension1=AoA  Table=CL  InternalRulePriority=Speed  RndMeth=Simplest
  1-D Lookup Table1 : Lookup_n-D  NumberOfTableDimensions=1  BreakpointsForDimension1=AoA  Table=CL  InternalRulePriority=Speed  RndMeth=Simplest
  Angle Conversion2 : aerolibconvert2/Angle Conversion  IU=rad  OU=deg
  Angle Conversion4 : aerolibconvert2/Angle Conversion  IU=rad  OU=deg
  Gain : Gain  Gain=-1
  Saturation1 : Saturate  UpperLimit=0.15  LowerLimit=-0.05  LinearizeAsGain=off
  Saturation2 : Saturate  UpperLimit=0.15  LowerLimit=-0.05  LinearizeAsGain=off
  CL : Outport
  CD : Outport  Port=2
  wires:
  Angle Conversion2/1 -> Saturation1/1
  Angle Conversion4/1 -> Saturation2/1
  1-D Lookup Table1/1 -> CD/1
  1-D Lookup Table/1 -> CL/1
  In1/1 -> Gain/1
  Saturation1/1 -> 1-D Lookup Table/1
  Saturation2/1 -> 1-D Lookup Table1/1
  Gain/1 -> Angle Conversion4/1, Angle Conversion2/1

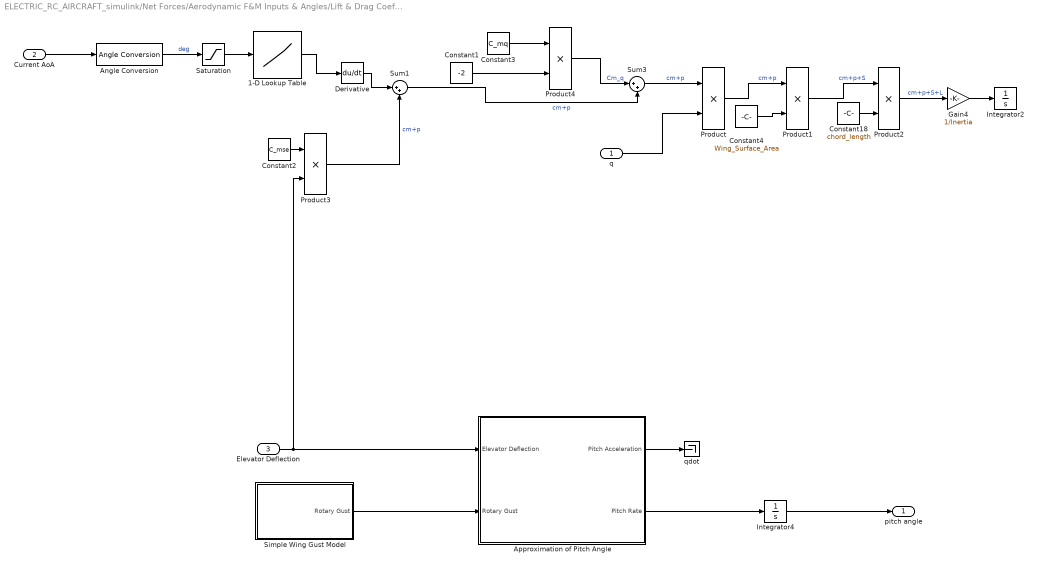
== system ELECTRIC_RC_AIRCRAFT_simulink/Net Forces/Aerodynamic F&M Inputs & Angles/Lift & Drag Coefficients/Pitch Angle Calculation ==
  q : Inport
  Current AoA : Inport  Port=2
  Elevator Deflection : Inport  Port=3
  1-D Lookup Table : Lookup_n-D  NumberOfTableDimensions=1  BreakpointsForDimension1=[-5 0 5 10]  Table=CM  InternalRulePriority=Speed  RndMeth=Simplest
  Angle Conversion : aerolibconvert2/Angle Conversion  IU=rad  OU=deg
  Approximation of Pitch Angle : Subsystem
  Constant1 : Constant  Value=-2
  Constant18 : Constant  Value=chord_length
  Constant2 : Constant  Value=C_mse
  Constant3 : Constant  Value=C_mq
  Constant4 : Constant  Value=Wing_Surface_Area
  Derivative : Derivative
  Gain4 : Gain  Gain=1/Inertia
  Integrator2 : Integrator
  Integrator4 : Integrator
  Product{,1..4} (5 alike) : Product
  Saturation : Saturate  UpperLimit=10  LowerLimit=-10  LinearizeAsGain=off
  Simple Wing Gust Model : Subsystem
  Sum1 : Sum  Inputs=|++
  Sum3 : Sum  Inputs=|++
  qdot : Terminator
  pitch angle : Outport
  wires:
  Product/1 -> Product1/1  "cm+p"
  Constant18/1 -> Product2/2
  Product1/1 -> Product2/1  "cm+p+S"
  Current AoA/1 -> Angle Conversion/1
  Constant4/1 -> Product1/2
  Gain4/1 -> Integrator2/1
  q/1 -> Product/2
  Saturation/1 -> 1-D Lookup Table/1
  Product2/1 -> Gain4/1  "cm+p+S+L"
  Angle Conversion/1 -> Saturation/1  "deg"
  1-D Lookup Table/1 -> Derivative/1
  Derivative/1 -> Sum1/1
  Sum1/1 -> Sum3/2  "cm+p"
  Constant1/1 -> Product4/2
  Product4/1 -> Sum3/1  "Cm_q"
  Constant2/1 -> Product3/1
  Product3/1 -> Sum1/2  "cm+p"
  Constant3/1 -> Product4/1
  Sum3/1 -> Product/1  "cm+p"
  Simple Wing Gust Model/1(Rotary Gust) -> Approximation of Pitch Angle/2(Rotary Gust)
  Elevator Deflection/1 -> Product3/2, Approximation of Pitch Angle/1(Elevator Deflection)
  Approximation of Pitch Angle/2(Pitch Rate) -> Integrator4/1
  Approximation of Pitch Angle/1(Pitch Acceleration) -> qdot/1
  Integrator4/1 -> pitch angle/1

== system ELECTRIC_RC_AIRCRAFT_simulink/Net Forces/Elevator Model System/Pitch Angle Calculation/Aircraft Dynamics Model ==
  Elevator Deflection d (rad) : Inport
  Rotary Gust qGust (rad/sec) : Inport  Port=2
  Gain6 : Gain  Gain=0.1  SaturateOnIntegerOverflow=on  OutDataTypeStr=Inherit: Same as input  ParamDataTypeStr=Inherit: Same as input
  Pitch Channel : Subsystem
  Scope : Scope
      settings: ActiveDisplayYMinimum=-3.8661690224856295  ActiveDisplayYMaximum=2.9706017130705988  DataLoggingVariableName=ScopeData8
  Sum : Sum  Inputs=|-+
  Pitch Accel qdot (rad/sec2) : Outport  InitialOutput=0  VectorParamsAs1DForOutWhenUnconnected=off
  Pitch Rate q (rad/sec) : Outport  Port=2  InitialOutput=0  VectorParamsAs1DForOutWhenUnconnected=off
  wires:
  Sum/1 -> Pitch Channel/1(Input)
  Elevator Deflection d (rad)/1 -> Gain6/1
  Pitch Channel/2(qdot) -> Scope/1, Pitch Accel qdot (rad/sec2)/1
  Gain6/1 -> Sum/2
  Pitch Channel/1(q) -> Pitch Rate q (rad/sec)/1
  Rotary Gust qGust (rad/sec)/1 -> Sum/1

== system ELECTRIC_RC_AIRCRAFT_simulink/Net Forces/Elevator Model System/Pitch Angle Calculation/Simple Wing Gust Model ==
  Band-Limited White Noise : simulink/Sources/Band-Limited White Noise  Cov=0.1  Ts=1/30  seed=[23341]
  Gain1 : Gain  Gain=0.05  SaturateOnIntegerOverflow=on  OutDataTypeStr=Inherit: Same as input  ParamDataTypeStr=Inherit: Same as input
  Gain3 : Gain  Gain=0  SaturateOnIntegerOverflow=on  OutDataTypeStr=Inherit: Same as input  ParamDataTypeStr=Inherit: Same as input
  Sum : Sum  Inputs=|++  InputSameDT=on  SaturateOnIntegerOverflow=on  OutDataTypeStr=Inherit: Same as first input
  Pitch Gust Accel. (qdotGust) : Outport  InitialOutput=0  VectorParamsAs1DForOutWhenUnconnected=off
  wires:
  Gain1/1 -> Sum/2
  Sum/1 -> Pitch Gust Accel. (qdotGust)/1
  Gain3/1 -> Sum/1, Gain1/1
  Band-Limited White Noise/1 -> Gain3/1

== system ELECTRIC_RC_AIRCRAFT_simulink/Net Forces/Aerodynamic F&M Inputs & Angles/Lift & Drag Coefficients/Pitch Angle Calculation/Approximation of Pitch Angle ==
  Elevator Deflection : Inport
  Rotary Gust : Inport  Port=2
  Gain6 : Gain  Gain=0.5  SaturateOnIntegerOverflow=on  OutDataTypeStr=Inherit: Same as input  ParamDataTypeStr=Inherit: Same as input
  Pitch Channel : Subsystem
  Sum : Sum  Inputs=|-+
  Pitch Acceleration : Outport  InitialOutput=0  VectorParamsAs1DForOutWhenUnconnected=off
  Pitch Rate : Outport  Port=2  InitialOutput=0  VectorParamsAs1DForOutWhenUnconnected=off
  wires:
  Sum/1 -> Pitch Channel/1(Input)
  Elevator Deflection/1 -> Gain6/1
  Rotary Gust/1 -> Sum/1
  Pitch Channel/2(Pitch Acceleration) -> Pitch Acceleration/1
  Gain6/1 -> Sum/2
  Pitch Channel/1(Pitch rate) -> Pitch Rate/1

== system ELECTRIC_RC_AIRCRAFT_simulink/Net Forces/Aerodynamic F&M Inputs & Angles/Lift & Drag Coefficients/Pitch Angle Calculation/Simple Wing Gust Model ==
  Band-Limited White Noise : simulink/Sources/Band-Limited White Noise  Cov=0.1  Ts=1/30  seed=[23341]
  Gain1 : Gain  Gain=0.05  SaturateOnIntegerOverflow=on  OutDataTypeStr=Inherit: Same as input  ParamDataTypeStr=Inherit: Same as input
  Gain3 : Gain  Gain=0  SaturateOnIntegerOverflow=on  OutDataTypeStr=Inherit: Same as input  ParamDataTypeStr=Inherit: Same as input
  Sum : Sum  Inputs=|++  InputSameDT=on  SaturateOnIntegerOverflow=on  OutDataTypeStr=Inherit: Same as first input
  Rotary Gust : Outport  InitialOutput=0  VectorParamsAs1DForOutWhenUnconnected=off
  wires:
  Gain1/1 -> Sum/2
  Sum/1 -> Rotary Gust/1
  Gain3/1 -> Sum/1, Gain1/1
  Band-Limited White Noise/1 -> Gain3/1

== system ELECTRIC_RC_AIRCRAFT_simulink/Net Forces/Elevator Model System/Pitch Angle Calculation/Aircraft Dynamics Model/Pitch Channel ==
  Input : Inport
  Gain : Gain  Gain=-0.772  SaturateOnIntegerOverflow=on  OutDataTypeStr=Inherit: Same as input  ParamDataTypeStr=Inherit: Same as input
  Integrate qdot : Integrator
  Sum : Sum  Inputs=|++  InputSameDT=on  SaturateOnIntegerOverflow=on  OutDataTypeStr=Inherit: Same as first input
  q : Outport  InitialOutput=0  VectorParamsAs1DForOutWhenUnconnected=off
  qdot : Outport  Port=2  InitialOutput=0  VectorParamsAs1DForOutWhenUnconnected=off
  wires:
  Sum/1 -> qdot/1, Integrate qdot/1
  Integrate qdot/1 -> Gain/1, q/1
  Gain/1 -> Sum/2
  Input/1 -> Sum/1

== system ELECTRIC_RC_AIRCRAFT_simulink/Net Forces/Aerodynamic F&M Inputs & Angles/Lift & Drag Coefficients/Pitch Angle Calculation/Approximation of Pitch Angle/Pitch Channel ==
  Input : Inport
  Gain : Gain  Gain=-0.772  SaturateOnIntegerOverflow=on  OutDataTypeStr=Inherit: Same as input  ParamDataTypeStr=Inherit: Same as input
  Integrate qdot : Integrator
  Sum : Sum  Inputs=|++  InputSameDT=on  SaturateOnIntegerOverflow=on  OutDataTypeStr=Inherit: Same as first input
  Pitch rate : Outport  InitialOutput=0  VectorParamsAs1DForOutWhenUnconnected=off
  Pitch Acceleration : Outport  Port=2  InitialOutput=0  VectorParamsAs1DForOutWhenUnconnected=off
  wires:
  Sum/1 -> Pitch Acceleration/1, Integrate qdot/1
  Integrate qdot/1 -> Gain/1, Pitch rate/1
  Gain/1 -> Sum/2
  Input/1 -> Sum/1
